simulink model "Task_C"  (R2022b)
settings: Solver=ode45  StartTime=0.0  StopTime=10.0  RelTol=1e-3
undefined symbols (not defined in the file): init, K_ctr, K_I
libraries: simulink_extras x5, simulink x1
settings Model: Creator=tumisangramotlhwa  LastModifiedBy=tumisangramotlhwa

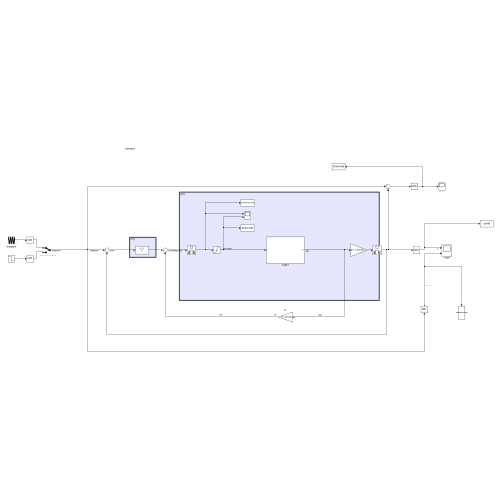
[thumbnail: Simulink's stored preview of the top-level diagram]
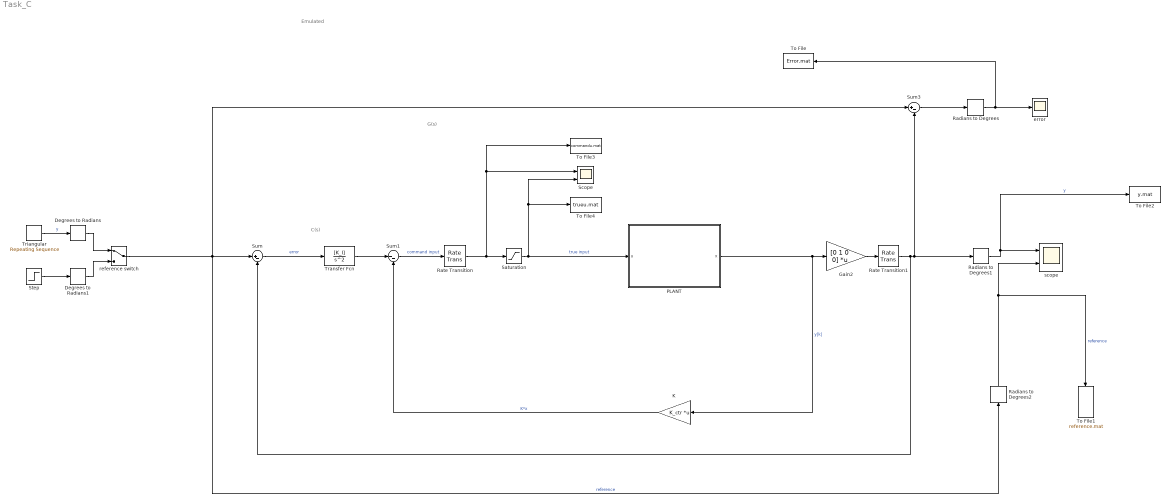
== system Task_C ==
  note: Emulated
  note: G(s)
  note: C(s)
  " Triangular" : simulink/Sources/Repeating Sequence  rep_seq_t=[0 2 4]  rep_seq_y=[45 15 45]
  Degrees to Radians : simulink_extras/Transformations/Degrees to Radians
  Degrees to Radians1 : simulink_extras/Transformations/Degrees to Radians
  Gain2 : Gain  Gain=[0 1 0 0]  Multiplication=Matrix(K*u) (u vector)
  K : Gain  Gain=K_ctr  Multiplication=Matrix(K*u) (u vector)
  PLANT : Subsystem
  Radians to Degrees : simulink_extras/Transformations/Radians to Degrees
  Radians to Degrees1 : simulink_extras/Transformations/Radians to Degrees
  Radians to Degrees2 : simulink_extras/Transformations/Radians to Degrees
  Rate Transition : RateTransition  OutPortSampleTime=1/50
  Rate Transition1 : RateTransition  OutPortSampleTime=1/50
  Saturation : Saturate  UpperLimit=6  LowerLimit=-6
  Scope : Scope  NumInputPorts=2
  Step : Step  Before=45  After=15  SampleTime=0
  Sum : Sum  Inputs=|+-
  Sum1 : Sum  Inputs=|--
  Sum3 : Sum  Inputs=|+-
  To File : ToFile  Filename=Error.mat  MatrixName=Error  SaveFormat=Timeseries
  To File1 : ToFile  Filename=reference.mat  MatrixName=reference  SaveFormat=Timeseries
  To File2 : ToFile  Filename=y.mat  MatrixName=y  SaveFormat=Timeseries
  To File3 : ToFile  Filename=commandu.mat  MatrixName=commandu  SaveFormat=Timeseries
  To File4 : ToFile  Filename=trueu.mat  MatrixName=trueu  SaveFormat=Timeseries
  Transfer Fcn : TransferFcn  Numerator=[K_I]  Denominator=[1 0 0]
  error : Scope
  reference switch : ManualSwitch
  scope : Scope  NumInputPorts=2
  wires:
  reference switch/1 -> Sum3/1, Sum/1, Radians to Degrees2/1  "reference"
  Step/1 -> Degrees to Radians1/1
  " Triangular"/1 -> Degrees to Radians/1  "y"
  Sum3/1 -> Radians to Degrees/1
  Radians to Degrees/1 -> error/1, To File/1
  Radians to Degrees1/1 -> scope/1, To File2/1  "y"
  Radians to Degrees2/1 -> scope/2, To File1/1  "reference"
  Sum/1 -> Transfer Fcn/1  "error"
  Saturation/1 -> To File4/1, Scope/2, PLANT/1(u)  "true input"
  Sum1/1 -> Rate Transition/1  "command input"
  K/1 -> Sum1/2  "K*x"
  Degrees to Radians/1 -> reference switch/1
  Degrees to Radians1/1 -> reference switch/2
  PLANT/1(x) -> Gain2/1, K/1  "y[k]"
  Transfer Fcn/1 -> Sum1/1
  Gain2/1 -> Rate Transition1/1
  Rate Transition1/1 -> Sum3/2, Radians to Degrees1/1, Sum/2
  Rate Transition/1 -> To File3/1, Scope/1, Saturation/1

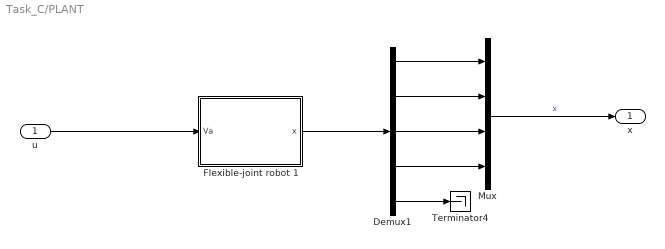
== system Task_C/PLANT ==
  u : Inport
  Demux1 : Demux  Outputs=5
  Flexible-joint robot 1 : Subsystem
      mask Display: image('$imagefile'); % Use "Edit Image" on toolstrip to change.
  Mux : Mux
  Terminator4 : Terminator
  x : Outport
  wires:
  Mux/1 -> x/1  "x"
  Demux1/4 -> Mux/4
  Flexible-joint robot 1/1(x) -> Demux1/1
  Demux1/3 -> Mux/3
  Demux1/2 -> Mux/2
  Demux1/1 -> Mux/1
  Demux1/5 -> Terminator4/1
  u/1 -> Flexible-joint robot 1/1(Va)

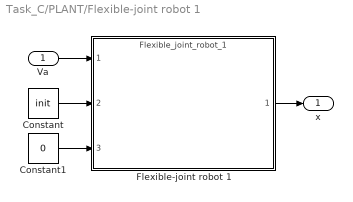
== system Task_C/PLANT/Flexible-joint robot 1 ==
  Va : Inport
  Constant : Constant  Value=init
  Constant1 : Constant  Value=0
  Flexible-joint robot 1 : ModelReference  ModelNameDialog=Flexible_joint_robot_1  ModelReferenceVersion=1.63  CopyOfModelProtected=on
  x : Outport
  wires:
  Constant/1 -> Flexible-joint robot 1/2
  Constant1/1 -> Flexible-joint robot 1/3
  Flexible-joint robot 1/1 -> x/1
  Va/1 -> Flexible-joint robot 1/1
